simulink model "local_sequencer_harness1"  (R2018b)
settings: Solver=FixedStepDiscrete  StartTime=0  StopTime=8  FixedStep=1  RelTol=1e-3
undefined symbols (not defined in the file or in its folder): eof, sigbuilder_block, sldvsubsys, StateFlowModeType
libraries: sldvlib x21, simulink x6, hdlsllib x4
(part 1 of 2)
settings Model: SldvGeneratedHarnessModel=TestUnitModel=local_sequencer|  Creator=hiterd  LastModifiedBy=gauthamsm
settings DataIOCC: SaveFormat=StructureWithTime
settings OptimizationCC: BlockReduction=off  ConditionallyExecuteInputs=off  DefaultParameterBehavior=Inlined  ExpressionFolding=off
settings DebuggingCC: InheritedTsInSrcMsg=none  LibraryContextMissingDiagnostic=none
settings SFSimCC: SimUseLocalCustomCode=off
settings RTWCC: RTWUseLocalCustomCode=off
settings ConfigComp: DVMode=PropertyProving  DVModelCoverageObjectives=MCDC  DVTestSuiteOptimization=CombinedObjectives (Nonlinear Extended)  DVDetectOutOfBounds=on  DVSaveExpectedOutput=on  DVDisplayReport=off

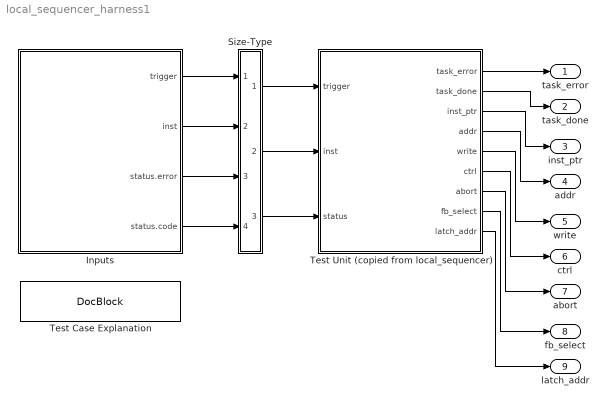
== system local_sequencer_harness1 ==
  Inputs : Subsystem  Tag=STV Subsys  LoadFcn=sigbuilder_block('load',[50 50 520 400 ]);  StartFcn=sigbuilder_block('start');  StopFcn=sigbuilder_block('stop');  ClipboardFcn=sigbuilder_block('clipboard');  mask(Sigbuilder block){tuvar=[0:10]}
      mask init:
      | if ~strcmp(get_param(bdroot(gcb),'SimulationStatus'),'stopped'),tuvar = sigbuilder_block('maskInit'); end
      settings: CopyFcn=sigbuilder_block('copy');  DeleteFcn=sigbuilder_block('delete');  ModelCloseFcn=sigbuilder_block('modelClose');  PreSaveFcn=sigbuilder_block('preSave');  PauseFcn=sigbuilder_block('pause');  ContinueFcn=sigbuilder_block('continue');  NameChangeFcn=sigbuilder_block('namechange');  OpenFcn=sigbuilder_block('open');  CloseFcn=sigbuilder_block('close');
      mask Display: plot(0, 0, 100, 100,[2, 2, 32, 32, 2], [68, 8, 8, 68, 68],[32, 2], [38, 38], [32, 19, 2],[53, 60, 44], [32, 17, 17, 2],[16, 16, 31, 31]);txt = getActiveGroup(gcbh);text(2, 100, txt,'verticalAlignment', 'top');
  Size-Type : Subsystem
  Test Case Explanation : simulink/Model-Wide Utilities/DocBlock  DocumentType=Text
  Test Unit (copied from local_sequencer) : Subsystem
  task_error : Outport  RequirementInfo={'linktype_rmi_slreq' 'local_sequencer_req.slreqx' '20' 'true' 'ERROR (local_sequencer_req#20)' '' ; 'linktype_rmi_slreq' 'local_sequencer_req.slreqx' '29' 'true' 'Error Signal Service Provided (local_sequencer_req#29)' '' } %GIDa_6eef222e_a01c_4fe0_8b87_beeef317aa57  OutDataTypeStr=boolean
  task_done : Outport  RequirementInfo={'linktype_rmi_slreq' 'local_sequencer_req.slreqx' '19' 'true' 'TASK_DONE (local_sequencer_req#19)' '' ; 'linktype_rmi_slreq' 'local_sequencer_req.slreqx' '30' 'true' 'Task Done Service Provided (local_sequencer_req#30)' '' } %GIDa_6d4806b7_f9de_4eac_b969_3ebe75b1e1cf  Port=2  OutDataTypeStr=boolean
  inst_ptr : Outport  RequirementInfo={'linktype_rmi_slreq' 'local_sequencer_req.slreqx' '32' 'true' 'Instruction Pointer Service Provided (local_sequencer_req#32)' '' } %GIDa_7b08b03b_531f_4ab3_8a58_ea9a3981e577  Port=3  OutDataTypeStr=task_inst_ptr_type
  addr : Outport  RequirementInfo={'linktype_rmi_slreq' 'local_sequencer_req.slreqx' '31' 'true' 'Task Memory Control Service Provided (local_sequencer_req#31)' '' } %GIDa_6cc3cc84_3630_4849_818a_038d439d27b6  Port=4  OutMin=[0]  OutDataTypeStr=task_memory_addr_type
  write : Outport  RequirementInfo={'linktype_rmi_slreq' 'local_sequencer_req.slreqx' '17' 'true' 'WRITE (local_sequencer_req#17)' '' ; 'linktype_rmi_slreq' 'local_sequencer_req.slreqx' '31' 'true' 'Task Memory Control Service Provided (local_sequencer_req#31)' '' } %GIDa_5bef7a76_c2bd_49e5_8166_1c241c27171b  Port=5  OutDataTypeStr=boolean
  ctrl : Outport  RequirementInfo={'linktype_rmi_slreq' 'local_sequencer_req.slreqx' '15' 'true' 'FETCH (local_sequencer_req#15)' '' ; 'linktype_rmi_slreq' 'local_sequencer_req.slreqx' '16' 'true' 'FB_EXECUTE (local_sequencer_req#16)' '' ; 'linktype_rmi_slreq' 'local_sequencer_req.slreqx' '17' 'true' 'WRITE (local_sequencer_req#17)' '' ; 'linktype_rmi_slreq' 'local_sequencer_req.slreqx' '18' 'true' 'FB_DONE (local_sequencer_req#18)' '' } %GIDa_e9a2eb4e_1730_43fc_aa4d_0d480ce4c4e5  Port=6  OutDataTypeStr=boolean
  abort : Outport  RequirementInfo={'linktype_rmi_slreq' 'local_sequencer_req.slreqx' '20' 'true' 'ERROR (local_sequencer_req#20)' '' } %GIDa_377a1d8d_f365_49c2_8f09_411d47a425b6  Port=7  OutDataTypeStr=boolean
  fb_select : Outport  RequirementInfo={'linktype_rmi_slreq' 'local_sequencer_req.slreqx' '33' 'true' 'Function Block Selection Service Provided (local_sequencer_req#33)' '' } %GIDa_773eebd4_072a_4a77_a6f5_8af07ffa45d2  Port=8  OutDataTypeStr=fb_select_type
  latch_addr : Outport  RequirementInfo={} %GIDa_0990d834_66a0_4e94_ab9b_9875cb70122a  Port=9  OutMin=[0]  OutDataTypeStr=boolean
  wires:
  Inputs/1(trigger) -> Size-Type/1(In1)
  Size-Type/1(Out1) -> Test Unit (copied from local_sequencer)/1(trigger)
  Inputs/2(inst) -> Size-Type/2(In2)
  Size-Type/2(Out2) -> Test Unit (copied from local_sequencer)/2(inst)
  Inputs/3(status.error) -> Size-Type/3(In5)
  Inputs/4(status.code) -> Size-Type/4(In6)
  Size-Type/3(Out3) -> Test Unit (copied from local_sequencer)/3(status)
  Test Unit (copied from local_sequencer)/1(task_error) -> task_error/1
  Test Unit (copied from local_sequencer)/2(task_done) -> task_done/1
  Test Unit (copied from local_sequencer)/3(inst_ptr) -> inst_ptr/1
  Test Unit (copied from local_sequencer)/4(addr) -> addr/1
  Test Unit (copied from local_sequencer)/5(write) -> write/1
  Test Unit (copied from local_sequencer)/6(ctrl) -> ctrl/1
  Test Unit (copied from local_sequencer)/7(abort) -> abort/1
  Test Unit (copied from local_sequencer)/8(fb_select) -> fb_select/1
  Test Unit (copied from local_sequencer)/9(latch_addr) -> latch_addr/1

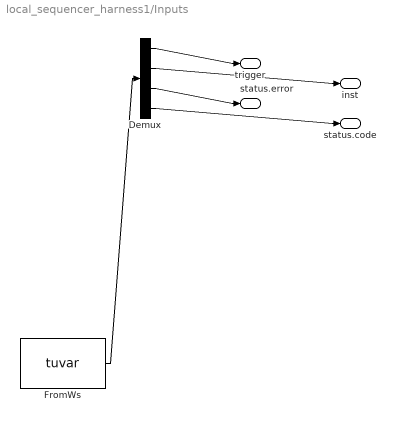
== system local_sequencer_harness1/Inputs ==
  Demux : Demux  Tag=STV Demux
  FromWs : FromWorkspace  Tag=STV FromWs  VariableName=tuvar  SampleTime=0
      SigBuilderData=|
      | dataSet(1).timeRange = [0 7]
      | dataSet(1).name = 'Counterexample 1'
      | dataSet(2).timeRange = [0 8]
      | dataSet(2).name = 'Counterexample 2'
      | sbobj.Name = 'Signal Builder'
      | sbobj.Groups(1).Name = 'Counterexample 1'
      | sbobj.Groups(1).Signals(1).Name = 'trigger'
      | sbobj.Groups(1).Signals(1).XData = [0 1 2 3 4 5 5 6 7]
      | sbobj.Groups(1).Signals(1).YData = [1 1 1 1 1 1 0 0 0]
      | sbobj.Groups(1).Signals(2).Name = 'inst'
      | sbobj.Groups(1).Signals(2).XData = [0 1 2 3 4 5 6 7]
      | sbobj.Groups(1).Signals(2).YData = [2147483646 2147483646 2147483646 2147483646 2147483646 2147483646 2147483646 2147483646]
      | sbobj.Groups(1).Signals(3).Name = 'status.error'
      | sbobj.Groups(1).Signals(3).XData = [0 1 2 3 3 4 5 5 6 7]
      | sbobj.Groups(1).Signals(3).YData = [0 0 0 0 1 1 1 0 0 0]
      | sbobj.Groups(1).Signals(4).Name = 'status.code'
      | sbobj.Groups(1).Signals(4).XData = [0 1 1 2 2 3 3 4 4 5 5 6 6 7]
      | sbobj.Groups(1).Signals(4).YData = [71303169 71303169 8388609 8388609 2227175425 2227175425 2164260864 2164260864 2235564032 2235564032 2239758337 2239758337 96468993 96468993]
      | sbobj.Groups(1).TimeRange = [0 7]
      | sbobj.Groups(2).Name = 'Counterexample 2'
      | sbobj.Groups(2).Signals(1).Name = 'trigger'
      | sbobj.Groups(2).Signals(1).XData = [0 1 2 3 4 5 5 6 7 7 8]
      | sbobj.Groups(2).Signals(1).YData = [1 1 1 1 1 1 0 0 0 1 1]
      | sbobj.Groups(2).Signals(2).Name = 'inst'
      | sbobj.Groups(2).Signals(2).XData = [0 1 2 3 4 5 6 7 8]
      | sbobj.Groups(2).Signals(2).YData = [2147483646 2147483646 2147483646 2147483646 2147483646 2147483646 2147483646 2147483646 2147483646]
      | sbobj.Groups(2).Signals(3).Name = 'status.error'
      | sbobj.Groups(2).Signals(3).XData = [0 1 2 3 3 4 5 5 6 7 8]
      | sbobj.Groups(2).Signals(3).YData = [0 0 0 0 1 1 1 0 0 0 0]
      | sbobj.Groups(2).Signals(4).Name = 'status.code'
      | sbobj.Groups(2).Signals(4).XData = [0 1 1 2 2 3 3 4 4 5 5 6 6 7 7 8]
      | sbobj.Groups(2).Signals(4).YData = [71303169 71303169 8388609 8388609 2227175425 2227175425 2164260865 2164260865 2235564033 2235564033 2239758337 2239758337 2243952640 2243952640 100663297 100663297]
      | sbobj.Groups(2).TimeRange = [0 8]
  trigger : Outport  Tag=STV Outport
  inst : Outport  Tag=STV Outport  Port=2
  status.error : Outport  Tag=STV Outport  Port=3
  status.code : Outport  Tag=STV Outport  Port=4
  wires:
  FromWs/1 -> Demux/1
  Demux/1 -> trigger/1
  Demux/2 -> inst/1
  Demux/3 -> status.error/1
  Demux/4 -> status.code/1

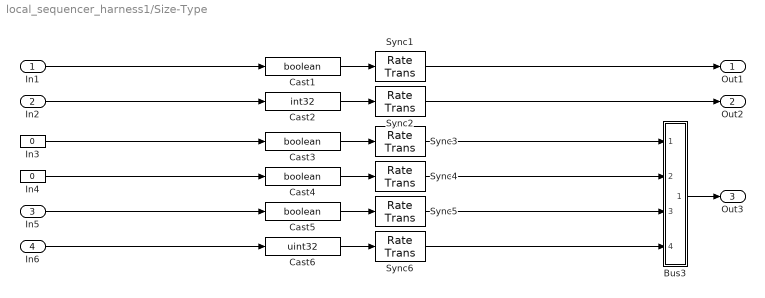
== system local_sequencer_harness1/Size-Type ==
  In1 : Inport
  In2 : Inport  Port=2
  In5 : Inport  Port=3
  In6 : Inport  Port=4
  Bus3 : Subsystem
  Cast{1,3..5} (4 alike) : DataTypeConversion  OutDataTypeStr=boolean  RndMeth=Nearest  SaturateOnIntegerOverflow=on
  Cast2 : DataTypeConversion  OutDataTypeStr=int32  RndMeth=Nearest  SaturateOnIntegerOverflow=on
  Cast6 : DataTypeConversion  OutDataTypeStr=uint32  RndMeth=Nearest  SaturateOnIntegerOverflow=on
  In3 : Constant  Value=0  OutDataTypeStr=double
  In4 : Constant  Value=0  OutDataTypeStr=double
  Sync{1..6} (6 alike) : RateTransition  OutPortSampleTime=[1,0]
  Out1 : Outport
  Out2 : Outport  Port=2
  Out3 : Outport  Port=3
  wires:
  In1/1 -> Cast1/1
  Cast1/1 -> Sync1/1
  Sync1/1 -> Out1/1
  In2/1 -> Cast2/1
  Cast2/1 -> Sync2/1
  Sync2/1 -> Out2/1
  In3/1 -> Cast3/1
  Cast3/1 -> Sync3/1
  In4/1 -> Cast4/1
  Cast4/1 -> Sync4/1
  In5/1 -> Cast5/1
  Cast5/1 -> Sync5/1
  In6/1 -> Cast6/1
  Cast6/1 -> Sync6/1
  Sync3/1 -> Bus3/1(status(1).done)
  Sync4/1 -> Bus3/2(status(1).busy)
  Sync5/1 -> Bus3/3(status(1).error)
  Sync6/1 -> Bus3/4(status(1).code)
  Bus3/1(Out) -> Out3/1

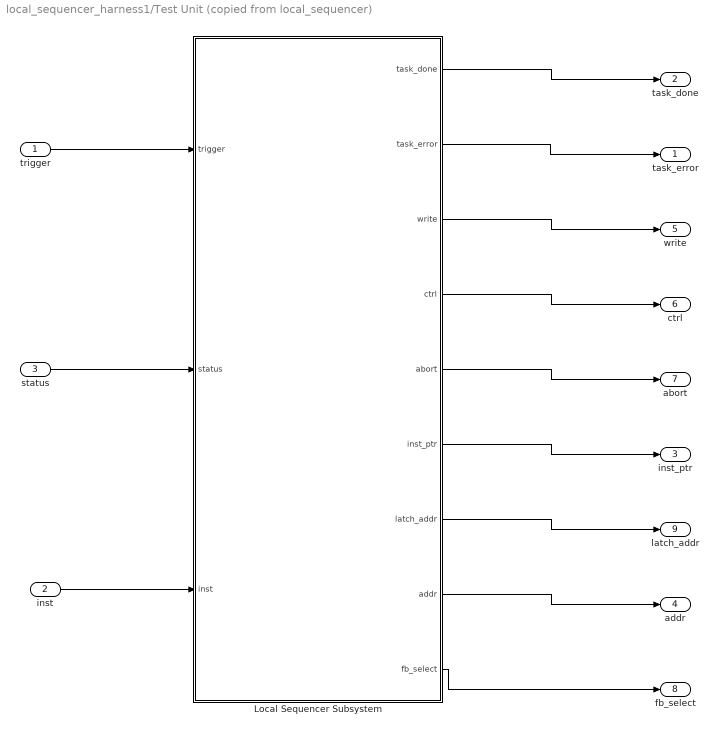
== system local_sequencer_harness1/Test Unit (copied from local_sequencer) ==
  trigger : Inport  RequirementInfo={'linktype_rmi_slreq' 'local_sequencer_req.slreqx' '1' 'true' 'Trigger Service Received (local_sequencer_req#1)' '' } %GIDa_ee1d0688_7702_4e59_8607_409a267b03c8  OutDataTypeStr=boolean  SampleTime=1
  inst : Inport  RequirementInfo={'linktype_rmi_slreq' 'local_sequencer_req.slreqx' '2' 'true' 'Instruction Service Received (local_sequencer_req#2)' '' } %GIDa_47f0b591_29ce_4c3a_8458_22a20f7cfe60  Port=2  OutDataTypeStr=task_inst_data_type  SampleTime=1
  status : Inport  RequirementInfo={'linktype_rmi_slreq' 'local_sequencer_req.slreqx' '3' 'true' 'Function Block Status Service Received (local_sequencer_req#3)' '' } %GIDa_5f43f148_b0c6_4574_8c0e_1a7e8a450581  Port=3  OutDataTypeStr=Bus: fb_status  SampleTime=1
  Local Sequencer Subsystem : Subsystem  RequirementInfo={} %GIDa_1bf9c4de_d1bc_41bc_89dd_bd5a58f40b8b
  task_error : Outport  RequirementInfo={'linktype_rmi_slreq' 'local_sequencer_req.slreqx' '20' 'true' 'ERROR (local_sequencer_req#20)' '' ; 'linktype_rmi_slreq' 'local_sequencer_req.slreqx' '29' 'true' 'Error Signal Service Provided (local_sequencer_req#29)' '' } %GIDa_20f58596_03f6_49ea_9ef8_6cf8984f0cae  OutDataTypeStr=boolean
  task_done : Outport  RequirementInfo={'linktype_rmi_slreq' 'local_sequencer_req.slreqx' '19' 'true' 'TASK_DONE (local_sequencer_req#19)' '' ; 'linktype_rmi_slreq' 'local_sequencer_req.slreqx' '30' 'true' 'Task Done Service Provided (local_sequencer_req#30)' '' } %GIDa_bf8ce283_f71f_479c_b035_26f3616a3704  Port=2  OutDataTypeStr=boolean
  inst_ptr : Outport  RequirementInfo={'linktype_rmi_slreq' 'local_sequencer_req.slreqx' '32' 'true' 'Instruction Pointer Service Provided (local_sequencer_req#32)' '' } %GIDa_0f6bf1a4_d050_45ca_8bf8_3a42e5078f97  Port=3  OutDataTypeStr=task_inst_ptr_type
  addr : Outport  RequirementInfo={'linktype_rmi_slreq' 'local_sequencer_req.slreqx' '31' 'true' 'Task Memory Control Service Provided (local_sequencer_req#31)' '' } %GIDa_98fe4c2c_df0f_4e0e_8fd6_d95b2a2e6c87  Port=4  OutMin=[0]  OutDataTypeStr=task_memory_addr_type
  write : Outport  RequirementInfo={'linktype_rmi_slreq' 'local_sequencer_req.slreqx' '17' 'true' 'WRITE (local_sequencer_req#17)' '' ; 'linktype_rmi_slreq' 'local_sequencer_req.slreqx' '31' 'true' 'Task Memory Control Service Provided (local_sequencer_req#31)' '' } %GIDa_17540029_023b_4499_94ff_6577575a4c02  Port=5  OutDataTypeStr=boolean
  ctrl : Outport  RequirementInfo={'linktype_rmi_slreq' 'local_sequencer_req.slreqx' '15' 'true' 'FETCH (local_sequencer_req#15)' '' ; 'linktype_rmi_slreq' 'local_sequencer_req.slreqx' '16' 'true' 'FB_EXECUTE (local_sequencer_req#16)' '' ; 'linktype_rmi_slreq' 'local_sequencer_req.slreqx' '17' 'true' 'WRITE (local_sequencer_req#17)' '' ; 'linktype_rmi_slreq' 'local_sequencer_req.slreqx' '18' 'true' 'FB_DONE (local_sequencer_req#18)' '' } %GIDa_b953f4cf_75e3_49f5_957d_136b7d9f114f  Port=6  OutDataTypeStr=boolean
  abort : Outport  RequirementInfo={'linktype_rmi_slreq' 'local_sequencer_req.slreqx' '20' 'true' 'ERROR (local_sequencer_req#20)' '' } %GIDa_64b414b4_42fd_4a02_80e3_9b85f133adaf  Port=7  OutDataTypeStr=boolean
  fb_select : Outport  RequirementInfo={'linktype_rmi_slreq' 'local_sequencer_req.slreqx' '33' 'true' 'Function Block Selection Service Provided (local_sequencer_req#33)' '' } %GIDa_ebf60c88_1429_4d3a_8715_399b1e400c0c  Port=8  OutDataTypeStr=fb_select_type
  latch_addr : Outport  RequirementInfo={} %GIDa_5b9c4f65_97de_40d7_b2b2_078d0fae9703  Port=9  OutMin=[0]  OutDataTypeStr=boolean
  wires:
  trigger/1 -> Local Sequencer Subsystem/1(trigger)
  status/1 -> Local Sequencer Subsystem/2(status)
  inst/1 -> Local Sequencer Subsystem/3(inst)
  Local Sequencer Subsystem/1(task_done) -> task_done/1
  Local Sequencer Subsystem/2(task_error) -> task_error/1
  Local Sequencer Subsystem/3(write) -> write/1
  Local Sequencer Subsystem/4(ctrl) -> ctrl/1
  Local Sequencer Subsystem/5(abort) -> abort/1
  Local Sequencer Subsystem/6(inst_ptr) -> inst_ptr/1
  Local Sequencer Subsystem/7(latch_addr) -> latch_addr/1
  Local Sequencer Subsystem/8(addr) -> addr/1
  Local Sequencer Subsystem/9(fb_select) -> fb_select/1

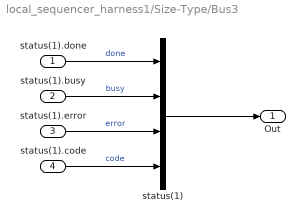
== system local_sequencer_harness1/Size-Type/Bus3 ==
  status(1).done : Inport
  status(1).busy : Inport  Port=2
  status(1).error : Inport  Port=3
  status(1).code : Inport  Port=4
  status(1) : BusCreator  Inputs=4  OutDataTypeStr=Bus: fb_status
  Out : Outport
  wires:
  status(1).done/1 -> status(1)/1  "done"
  status(1).busy/1 -> status(1)/2  "busy"
  status(1).error/1 -> status(1)/3  "error"
  status(1).code/1 -> status(1)/4  "code"
  status(1)/1 -> Out/1

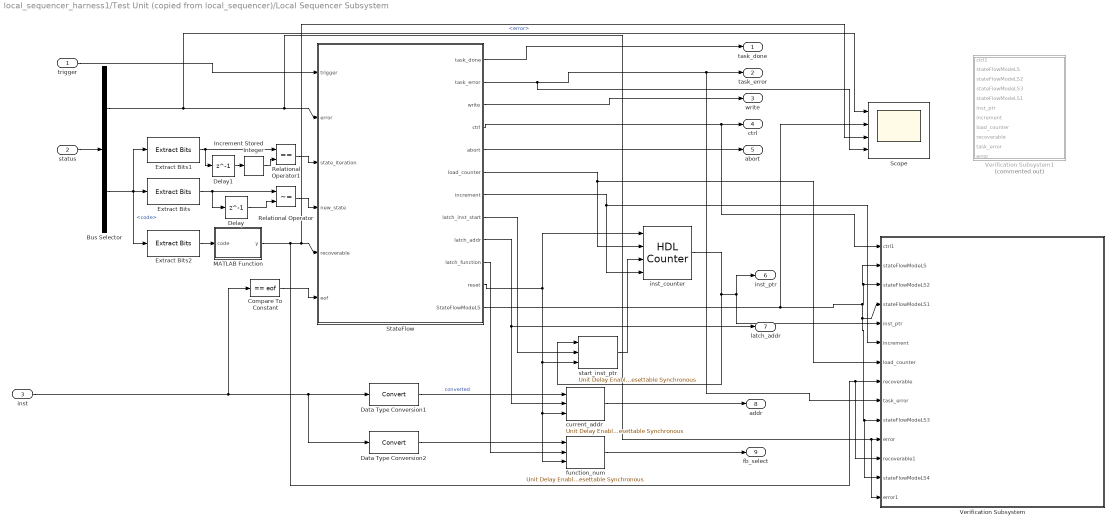
== system local_sequencer_harness1/Test Unit (copied from local_sequencer)/Local Sequencer Subsystem ==
  trigger : Inport  RequirementInfo={} %GIDa_667813c0_2ce9_40e6_9192_d23a19fa8e60
  status : Inport  RequirementInfo={} %GIDa_9f922e78_e05f_4ac9_a2b3_e973c3d7ad29  Port=2
  inst : Inport  RequirementInfo={} %GIDa_4c36c994_e89b_42c1_b8ba_4a193efc4b8e  Port=3
  Bus Selector : BusSelector  RequirementInfo={} %GIDa_79b6253a_0006_455f_9c58_eb6258196a1d  OutputSignals=error,code
  Compare To Constant : simulink/Logic and Bit Operations/Compare To Constant  RequirementInfo={'linktype_rmi_slreq' 'local_sequencer_req.slreqx' '7' 'true' 'End of File Determination (local_sequencer_req#7)' '' } %GIDa_d4bef37c_6deb_46bc_b5d5_b2c59b772020  relop===  const=eof  OutDataTypeStr=boolean
  Data Type Conversion1 : DataTypeConversion  RequirementInfo={'linktype_rmi_slreq' 'local_sequencer_req.slreqx' '34' 'true' 'Conversion of Data Input (local_sequencer_req#34)' '' } %GIDa_3a8a9ada_8e73_438c_a14d_fd8a1bd1786e
  Data Type Conversion2 : DataTypeConversion  RequirementInfo={'linktype_rmi_slreq' 'local_sequencer_req.slreqx' '34' 'true' 'Conversion of Data Input (local_sequencer_req#34)' '' } %GIDa_a57cdd45_237b_4637_96ce_ae33a3fb69d7
  Delay : Delay  RequirementInfo={'linktype_rmi_slreq' 'local_sequencer_req.slreqx' '5' 'true' 'Super State Change Detection (local_sequencer_req#5)' '' } %GIDa_45c36634_f8e4_4883_a8b8_e675ae30925e  DelayLength=1
  Delay1 : Delay  RequirementInfo={'linktype_rmi_slreq' 'local_sequencer_req.slreqx' '4' 'true' 'Super State Iteration Detection (local_sequencer_req#4)' '' } %GIDa_6506c89b_1702_47b1_a15e_211730d3d040  DelayLength=1
  Extract Bits : simulink/Logic and Bit Operations/Extract Bits  RequirementInfo={'linktype_rmi_slreq' 'local_sequencer_req.slreqx' '5' 'true' 'Super State Change Detection (local_sequencer_req#5)' '' } %GIDa_a09b6f6c_4604_4977_b275_4d844021750a  bitsToExtract=Range starting with most significant bit  numBits=4  bitIdxRange=[0 7]  outScalingMode=Treat bit field as an integer
      settings: SourceProductName=Simulink
  Extract Bits1 : simulink/Logic and Bit Operations/Extract Bits  RequirementInfo={'linktype_rmi_slreq' 'local_sequencer_req.slreqx' '4' 'true' 'Super State Iteration Detection (local_sequencer_req#4)' '' } %GIDa_e2105eee_930a_4cdf_b252_ae460803f0fd  bitsToExtract=Range of bits  numBits=4  bitIdxRange=[22 27]  outScalingMode=Treat bit field as an integer
      settings: SourceProductName=Simulink
  Extract Bits2 : simulink/Logic and Bit Operations/Extract Bits  RequirementInfo={'linktype_rmi_slreq' 'local_sequencer_req.slreqx' '6' 'true' 'Error Recovery Determination (local_sequencer_req#6)' '' } %GIDa_b560e2a3_a7f1_476c_8b2a_ffbd10a00e53  bitsToExtract=Range ending with least significant bit  numBits=22  bitIdxRange=[22 27]  outScalingMode=Treat bit field as an integer
      settings: SourceProductName=Simulink
  Increment Stored Integer : simulink/Additional Math & Discrete/Additional Math: Increment - Decrement/Increment Stored Integer  RequirementInfo={'linktype_rmi_slreq' 'local_sequencer_req.slreqx' '4' 'true' 'Super State Iteration Detection (local_sequencer_req#4)' '' } %GIDa_7ee8b49c_7e9e_43d6_94a5_684ad1a7ac3c
      settings: SourceProductName=Simulink
  MATLAB Function : MATLAB Function  RequirementInfo={'linktype_rmi_slreq' 'local_sequencer_req.slreqx' '6' 'true' 'Error Recovery Determination (local_sequencer_req#6)' '' } %GIDa_66948775_d3bd_4a51_9bc7_416a7d662e0f  TreatAsAtomicUnit=on
  Relational Operator : RelationalOperator  RequirementInfo={'linktype_rmi_slreq' 'local_sequencer_req.slreqx' '5' 'true' 'Super State Change Detection (local_sequencer_req#5)' '' } %GIDa_e58a5a39_9204_403d_bf5d_efec21faad89  Operator=~=  OutDataTypeStr=boolean  RndMeth=Nearest
  Relational Operator1 : RelationalOperator  RequirementInfo={'linktype_rmi_slreq' 'local_sequencer_req.slreqx' '4' 'true' 'Super State Iteration Detection (local_sequencer_req#4)' '' } %GIDa_773bf6c2_074e_418a_ba1a_320df8c963b4  Operator===  OutDataTypeStr=boolean  RndMeth=Nearest
  Scope : Scope  NumInputPorts=4
      settings: RequirementInfo={} %GIDa_a31c3830_a24c_4eea_be79_7702308a54d4
  StateFlow : Stateflow chart  RequirementInfo={'linktype_rmi_slreq' 'local_sequencer_req.slreqx' '12' 'true' 'Controller Super States (local_sequencer_req#12)' '' } %GIDa_024dda5f_4f1f_4977_87f0_8beb7680ab0a  TreatAsAtomicUnit=on
  Verification Subsystem : Subsystem  Tag=VerificationSubsystem  RequirementInfo={} %GIDa_838dcf04_7b59_4d43_9019_59a44524fb9a  DisableCoverage=on  LoadFcn=sldvsubsys('check')  TreatAsAtomicUnit=on  SimViewingDevice=on  mask(VerificationSubsystem){}
      mask init:
      | sldvsubsys('maskInit');
      settings: CopyFcn=sldvsubsys('copy');  OpenFcn=open_system(gcb,'force');
      settings: PreSaveFcn=|
      | set_param(gcb,'SimViewingDevice','on');
      | sldvsubsys('check');
      mask Help: helpview(fullfile(docroot,'toolbox','sldv','sldv.map'),'verificationsubsystem')
      mask Display: image(imread('sldvicon_versubsys.png','BackGroundColor',[1 1 1]),'center');
  Verification Subsystem1 : Subsystem  Tag=VerificationSubsystem  RequirementInfo={} %GIDa_73cb3161_c03e_414d_bb3b_35ff3da55f89  Commented=on  DisableCoverage=on  LoadFcn=sldvsubsys('check')  TreatAsAtomicUnit=on  SimViewingDevice=on  mask(VerificationSubsystem){}
      mask init:
      | sldvsubsys('maskInit');
      settings: CopyFcn=sldvsubsys('copy');  OpenFcn=open_system(gcb,'force');
      settings: PreSaveFcn=|
      | set_param(gcb,'SimViewingDevice','on');
      | sldvsubsys('check');
      mask Help: helpview(fullfile(docroot,'toolbox','sldv','sldv.map'),'verificationsubsystem')
      mask Display: image(imread('sldvicon_versubsys.png','BackGroundColor',[1 1 1]),'center');
  current_addr : hdlsllib/Discrete/Unit Delay Enabled Resettable Synchronous  RequirementInfo={'linktype_rmi_slreq' 'local_sequencer_req.slreqx' '11' 'true' 'Current Address Register (local_sequencer_req#11)' '' } %GIDa_563c094f_6702_4153_896a_e0e79255b215  InitialCondition=0  SampleTime=-1
      settings: SourceProductName=HDL Coder  SourceProductBaseCode=HD
  function_num : hdlsllib/Discrete/Unit Delay Enabled Resettable Synchronous  RequirementInfo={'linktype_rmi_slreq' 'local_sequencer_req.slreqx' '8' 'true' 'Function Number Register (local_sequencer_req#8)' '' } %GIDa_966114bc_cb8e_417e_b29d_e0445db8d5d9  InitialCondition=0  SampleTime=-1
      settings: SourceProductName=HDL Coder  SourceProductBaseCode=HD
  inst_counter : hdlsllib/Sources/HDL Counter  RequirementInfo={'linktype_rmi_slreq' 'local_sequencer_req.slreqx' '10' 'true' 'Instruction Counter (local_sequencer_req#10)' '' } %GIDa_defabc86_250d_4a18_b0b1_c3bf708ae8ef  CountType=Free running  CountInit=0  CountStep=1  CountMax=25  CountFromType=Initial value  CountFrom=0  CountResetPort=on  CountLoadPort=on  CountEnbPort=on  CountDirPort=off  CountDataType=Unsigned  CountWordLen=32  CountFracLen=0  CountSampTime=1
      settings: SourceProductBaseCode=HD
  start_inst_ptr : hdlsllib/Discrete/Unit Delay Enabled Resettable Synchronous  RequirementInfo={'linktype_rmi_slreq' 'local_sequencer_req.slreqx' '9' 'true' 'Start Instruction Pointer Register (local_sequencer_req#9)' '' } %GIDa_aaa9132d_cf81_4cca_ae88_9fa712b7ddec  InitialCondition=0  SampleTime=-1
      settings: SourceProductName=HDL Coder  SourceProductBaseCode=HD
  task_done : Outport  RequirementInfo={} %GIDa_60169851_d1f8_4054_83f8_3a56cf840165
  task_error : Outport  RequirementInfo={} %GIDa_5efbc127_0fad_4743_88d8_48387155e0aa  Port=2
  write : Outport  RequirementInfo={} %GIDa_a41ba5f4_8ba0_4949_8978_bbcfcaae8be3  Port=3
  ctrl : Outport  RequirementInfo={} %GIDa_2ac6603d_f9d3_4fa3_8391_63091cb403f2  Port=4
  abort : Outport  RequirementInfo={} %GIDa_76ad2b85_6a3f_4b60_a575_66190255e4d6  Port=5
  inst_ptr : Outport  RequirementInfo={} %GIDa_93e88be8_92b1_4795_b847_f82d81a6b850  Port=6
  latch_addr : Outport  RequirementInfo={} %GIDa_7a272877_8229_44a5_bbef_389013ad2e48  Port=7
  addr : Outport  RequirementInfo={} %GIDa_458cb3b4_2944_4610_af65_cc656e5cadff  Port=8
  fb_select : Outport  RequirementInfo={} %GIDa_946b26ee_232b_42dd_b12d_200ca52a7a09  Port=9
  wires:
  StateFlow/12(StateFlowModeLS) -> Verification Subsystem/2(stateFlowModeLS), Verification Subsystem/3(stateFlowModeLS2), Verification Subsystem/4(stateFlowModeLS1), Verification Subsystem/10(stateFlowModeLS3), Verification Subsystem/13(stateFlowModeLS4), Scope/2
  StateFlow/3(write) -> write/1
  current_addr/1 -> addr/1
  StateFlow/4(ctrl) -> ctrl/1, Verification Subsystem/1(ctrl1)
  StateFlow/1(task_done) -> task_done/1
  trigger/1 -> StateFlow/1(trigger)
  Extract Bits/1 -> Delay/1, Relational Operator/1
  MATLAB Function/1(y) -> StateFlow/5(recoverable), Scope/3, Verification Subsystem/8(recoverable), Verification Subsystem/12(recoverable1)
  StateFlow/10(latch_function) -> function_num/2
  Data Type Conversion2/1 -> function_num/1
  Relational Operator1/1 -> StateFlow/3(state_iteration)
  Delay/1 -> Relational Operator/2
  StateFlow/2(task_error) -> task_error/1, Verification Subsystem/9(task_error), Scope/4
  function_num/1 -> fb_select/1
  inst/1 -> Compare To Constant/1, Data Type Conversion2/1, Data Type Conversion1/1
  Compare To Constant/1 -> StateFlow/6(eof)
  Relational Operator/1 -> StateFlow/4(new_state)
  Bus Selector/1 -> StateFlow/2(error), Verification Subsystem/11(error), Verification Subsystem/14(error1), Scope/1  "<error>"
  inst_counter/1 -> start_inst_ptr/1, inst_ptr/1, Verification Subsystem/5(inst_ptr)
  Increment Stored Integer/1 -> Relational Operator1/2
  Delay1/1 -> Increment Stored Integer/1
  StateFlow/5(abort) -> abort/1
  Extract Bits1/1 -> Relational Operator1/1, Delay1/1
  Extract Bits2/1 -> MATLAB Function/1(code)
  Bus Selector/2 -> Extract Bits/1, Extract Bits1/1, Extract Bits2/1  "<code>"
  StateFlow/6(load_counter) -> inst_counter/2, Verification Subsystem/7(load_counter)
  StateFlow/11(reset) -> inst_counter/1, start_inst_ptr/3, current_addr/3, function_num/3
  start_inst_ptr/1 -> inst_counter/3
  Data Type Conversion1/1 -> current_addr/1  "converted"
  status/1 -> Bus Selector/1
  StateFlow/7(increment) -> inst_counter/4, Verification Subsystem/6(increment)
  StateFlow/8(latch_inst_start) -> start_inst_ptr/2
  StateFlow/9(latch_addr) -> current_addr/2, latch_addr/1

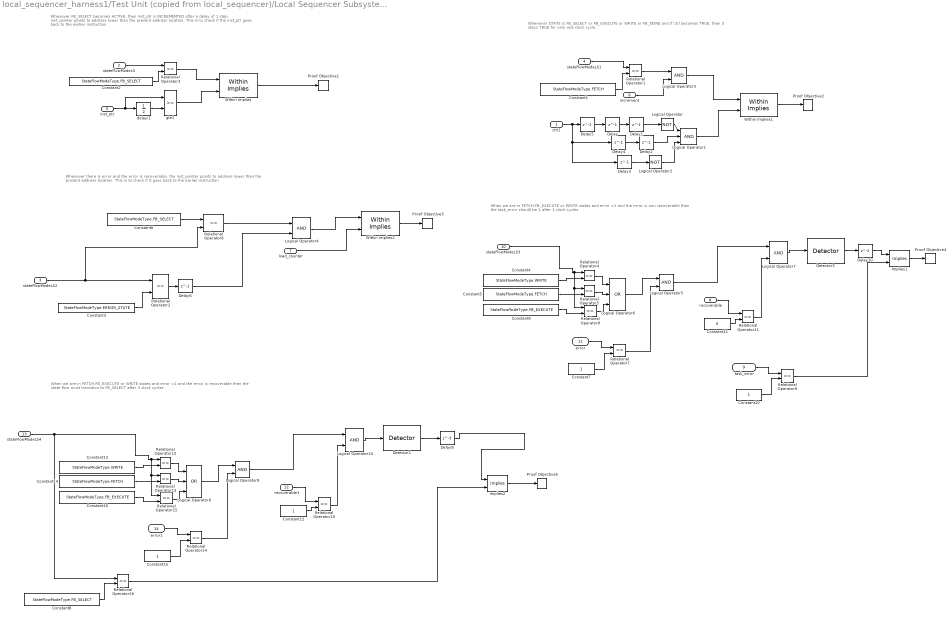
== system local_sequencer_harness1/Test Unit (copied from local_sequencer)/Local Sequencer Subsystem/Verification Subsystem ==
  note: When we are in FETCH,FB_EXECUTE or WRITE states and error =1 and the error is
      | recoverable then the state flow must transition to FB_SELECT after 3 clock cycles
  note: When we are in FETCH,FB_EXECUTE or WRITE states and error =1 and the error is non
      | recoverable then the task_error should be 1 after 2 clock cycles
  note: Whenever there is error and the error is recoverable, the inst_pointer points to address lower than the present address location. This is to check if it goes back to the earlier instruction
  note: Whenever STATE is FB_SELECT or FB_EXECUTE or WRITE or FB_DONE and if ctrl becomes TRUE, then it stays TRUE for only one clock cycle.
  note: Whenever FB_SELECT becomes ACTIVE, then inst_ptr is INCREMENTED after a delay of 1 step. inst_pointer points to address lower than the present address location. This is to check if the inst_ptr goes back to the earlier instruction
  ctrl1 : Inport  RequirementInfo={} %GIDa_2aa84e78_773c_4371_ae03_7363d7f38b64
  stateFlowModeLS : Inport  RequirementInfo={} %GIDa_cd1fa512_6795_43c1_a135_e70df5671345  Port=2  OutDataTypeStr=Enum: StateFlowModeType
  stateFlowModeLS2 : Inport  RequirementInfo={} %GIDa_3976201f_7908_44e8_8b3d_db7ce0af8161  Port=3  OutDataTypeStr=Enum: StateFlowModeType
  stateFlowModeLS1 : Inport  RequirementInfo={} %GIDa_58db11b1_1192_4008_8626_1d311f41fd79  Port=4  OutDataTypeStr=Enum: StateFlowModeType
  inst_ptr : Inport  RequirementInfo={} %GIDa_2b709768_3968_4a77_850c_0663ae289538  Port=5
  increment : Inport  RequirementInfo={} %GIDa_12b0bac8_6436_470f_99c5_ea1d75505bb8  Port=6
  load_counter : Inport  RequirementInfo={} %GIDa_d9eb1b57_669b_4c68_bafa_0f99cb4b8103  Port=7
  recoverable : Inport  RequirementInfo={} %GIDa_e4625633_5461_41a2_94bc_72442730136b  Port=8
  task_error : Inport  RequirementInfo={} %GIDa_cec4d3ba_40cf_4886_86fe_07ac90cae5b8  Port=9
  stateFlowModeLS3 : Inport  RequirementInfo={} %GIDa_c7061a7e_edfd_4dbe_80c8_d50c8470702e  Port=10  OutDataTypeStr=Enum: StateFlowModeType
  error : Inport  RequirementInfo={} %GIDa_b8bf48eb_8eb6_416e_ac24_17b4a0747917  Port=11
  recoverable1 : Inport  RequirementInfo={} %GIDa_6e7cca76_8046_47a7_bf72_a71fcb7542f0  Port=12
  stateFlowModeLS4 : Inport  RequirementInfo={} %GIDa_78b59d9b_505a_48a0_9be0_3dce6eb33108  Port=13  OutDataTypeStr=Enum: StateFlowModeType
  error1 : Inport  RequirementInfo={} %GIDa_60759bef_da0f_4b65_ab82_243b85aad350  Port=14
  Constant1 : Constant  RequirementInfo={} %GIDa_2f9b468e_86d5_4e67_b9d8_8570e8207cb9  Value=StateFlowModeType.FETCH
  Constant10 : Constant  RequirementInfo={} %GIDa_67375268_cc36_4cef_9a35_4af1b0917351
  Constant11 : Constant  RequirementInfo={} %GIDa_d249d429_5dab_46a5_ae30_b70515e1066b  Value=0
  Constant12 : Constant  RequirementInfo={} %GIDa_5e4e935c_c05b_470f_a371_33978611d8fb
  Constant13 : Constant  RequirementInfo={} %GIDa_253d0253_5ab4_4aa5_8c7d_2511dde3576a  Value=StateFlowModeType.WRITE
  Constant14 : Constant  RequirementInfo={} %GIDa_27c3072a_ad64_4193_8e57_068ee4e66af4  Value=StateFlowModeType.FETCH
  Constant15 : Constant  RequirementInfo={} %GIDa_3e0e1f5f_6b74_4bf1_a744_9088ebb3dfc4
  Constant16 : Constant  RequirementInfo={} %GIDa_fa8efd79_c799_4a6f_bdb6_1ef59b41cd93  Value=StateFlowModeType.FB_EXECUTE
  Constant2 : Constant  RequirementInfo={} %GIDa_5cb0de8b_a4d2_44b1_bb00_25cedf8883be  Value=StateFlowModeType.FB_SELECT
  Constant3 : Constant  RequirementInfo={} %GIDa_4c250295_da12_4c27_8ee3_9a2df8860d79  Value=StateFlowModeType.ERROR_STATE
  Constant4 : Constant  RequirementInfo={} %GIDa_2a0a2a41_61dc_4491_be58_822443834d8e  Value=StateFlowModeType.WRITE
  Constant5 : Constant  RequirementInfo={} %GIDa_362bda9a_a883_4331_93da_040566b8034c  Value=StateFlowModeType.FETCH
  Constant6 : Constant  RequirementInfo={} %GIDa_80f926aa_74f9_438f_a7de_40768c0b7c3b  Value=StateFlowModeType.FB_SELECT
  Constant7 : Constant  RequirementInfo={} %GIDa_bc8b03f5_f384_4a51_be3b_76328105cdb5
  Constant8 : Constant  RequirementInfo={} %GIDa_9b5bf724_cca9_4760_8981_bb49b685bd29  Value=StateFlowModeType.FB_SELECT
  Constant9 : Constant  RequirementInfo={} %GIDa_6af35a12_229c_4180_8d91_2e416acf6d9d  Value=StateFlowModeType.FB_EXECUTE
  Delay : Delay  RequirementInfo={} %GIDa_ce1a188c_ad47_4410_aca7_c02cd954dce1  DelayLength=1  InitialCondition=0
  Delay1 : Delay  RequirementInfo={} %GIDa_1362c001_f3eb_4d49_bb9c_0e94ad972754  DelayLength=1  InitialCondition=0
  Delay10 : Delay  RequirementInfo={} %GIDa_f01116f0_a0ee_44c9_b379_c02e42b855df  InitialCondition=0
  Delay2 : Delay  RequirementInfo={} %GIDa_1d4055f3_627a_43d5_8e73_8811762443c8  DelayLength=1  InitialCondition=0
  Delay3 : Delay  RequirementInfo={} %GIDa_ff1dd165_ed2d_4858_8b39_a6cd76526871  DelayLength=1  InitialCondition=0
  Delay4 : Delay  RequirementInfo={} %GIDa_c44a1d18_3025_443b_b4c5_471a8ae38f90  DelayLength=1  InitialCondition=0
  Delay5 : Delay  RequirementInfo={} %GIDa_9d77ba82_1771_4fe8_9992_2c0506f2e4b3  DelayLength=1  InitialCondition=0
  Delay6 : Delay  RequirementInfo={} %GIDa_71ec1c03_be14_4fbb_8dbf_80ce0c9cafb7  DelayLength=1  InitialCondition=0
  Delay8 : Delay  RequirementInfo={} %GIDa_c14d562a_418c_4025_9036_cae0ced13188  DelayLength=3  InitialCondition=0
  Detector1 : sldvlib/Temporal Operators/Detector  RequirementInfo={} %GIDa_8af342df_2d87_4d05_b53f_57649a8bece8  reset=off  typ=Synchronized  in_hold=1  delay=0  out_hold=5
      settings: SourceProductName=Simulink Design Verifier  SourceProductBaseCode=DV
  Detector3 : sldvlib/Temporal Operators/Detector  RequirementInfo={} %GIDa_24b06946_3181_402f_85ff_b2b774b0b6eb  reset=off  typ=Synchronized  in_hold=1  delay=0  out_hold=5
      settings: SourceProductName=Simulink Design Verifier  SourceProductBaseCode=DV
  Implies1 : sldvlib/Verification Utilities/Implies  RequirementInfo={} %GIDa_1c89ca27_fa5c_41ad_b908_4e82d2b3e8af
      settings: SourceProductName=Simulink Design Verifier  SourceProductBaseCode=DV
  Implies2 : sldvlib/Verification Utilities/Implies  RequirementInfo={} %GIDa_cbb2abe0_215a_4d24_ad95_12f29e4fb3c4
      settings: SourceProductName=Simulink Design Verifier  SourceProductBaseCode=DV
  Logical Operator : Logic  RequirementInfo={} %GIDa_61ff7ee5_b755_4f1a_91d7_94c52c251ca9  Operator=NOT  AllPortsSameDT=off  OutDataTypeStr=boolean
  Logical Operator1 : Logic  RequirementInfo={} %GIDa_3846ab15_8dd9_4095_b066_9fbc2776fd2e  Inputs=3  AllPortsSameDT=off  OutDataTypeStr=boolean
  Logical Operator10 : Logic  RequirementInfo={} %GIDa_b068508d_63f7_4024_a118_473cbfd4dbe4  AllPortsSameDT=off  OutDataTypeStr=boolean
  Logical Operator2 : Logic  RequirementInfo={} %GIDa_dc10462a_cf28_4017_82d4_4c6ffab9c4b8  Operator=NOT  AllPortsSameDT=off  OutDataTypeStr=boolean
  Logical Operator3 : Logic  RequirementInfo={} %GIDa_80b61834_e5e1_4893_b336_050aa4a3ce76  AllPortsSameDT=off  OutDataTypeStr=boolean
  Logical Operator4 : Logic  RequirementInfo={} %GIDa_3e32758b_ac4a_4dd0_b065_fe585041840a  AllPortsSameDT=off  OutDataTypeStr=boolean
  Logical Operator5 : Logic  RequirementInfo={} %GIDa_682725ea_3691_4e10_bf23_17cc8cf0e81c  AllPortsSameDT=off  OutDataTypeStr=boolean
  Logical Operator6 : Logic  RequirementInfo={} %GIDa_1a223ff8_058f_4edb_b86b_84cde330ac7a  Operator=OR  Inputs=3  AllPortsSameDT=off  OutDataTypeStr=boolean
  Logical Operator7 : Logic  RequirementInfo={} %GIDa_75707b2c_6c6f_4edb_b2e7_a30f65390c2f  AllPortsSameDT=off  OutDataTypeStr=boolean
  Logical Operator8 : Logic  RequirementInfo={} %GIDa_911bdfc3_0d8b_45dd_88b7_061381ed9f8d  AllPortsSameDT=off  OutDataTypeStr=boolean
  Logical Operator9 : Logic  RequirementInfo={} %GIDa_70ebfe4b_f92b_47a5_8eb3_0e675cff94de  Operator=OR  Inputs=3  AllPortsSameDT=off  OutDataTypeStr=boolean
  Proof Objective1 : sldvlib/Objectives and Constraints/Proof Objective  RequirementInfo={} %GIDa_7112df57_b338_4d19_9635_c3797f705c7b  enabled=on  customAVTBlockType=Proof Objective  intervals=true  dispValues=on  outEnabled=off  enableStopSim=off
      settings: AttributesFormatString=%<intervals>  SourceProductName=Simulink Design Verifier  SourceProductBaseCode=DV
  Proof Objective2 : sldvlib/Objectives and Constraints/Proof Objective  RequirementInfo={} %GIDa_4dbc438c_3680_4936_b3eb_536ccf53019f  enabled=on  customAVTBlockType=Proof Objective  intervals=true  dispValues=on  outEnabled=off  enableStopSim=off
      settings: AttributesFormatString=%<intervals>  SourceProductName=Simulink Design Verifier  SourceProductBaseCode=DV
  Proof Objective3 : sldvlib/Objectives and Constraints/Proof Objective  RequirementInfo={} %GIDa_0aa2b519_c2b4_452d_a934_518c9f2c2a78  enabled=on  customAVTBlockType=Proof Objective  intervals=true  dispValues=on  outEnabled=off  enableStopSim=off
      settings: AttributesFormatString=%<intervals>  SourceProductName=Simulink Design Verifier  SourceProductBaseCode=DV
  Proof Objective4 : sldvlib/Objectives and Constraints/Proof Objective  RequirementInfo={} %GIDa_251bef15_81a8_4130_b8c1_53605189bafa  enabled=on  customAVTBlockType=Proof Objective  intervals=true  dispValues=on  outEnabled=off  enableStopSim=off
      settings: AttributesFormatString=%<intervals>  SourceProductName=Simulink Design Verifier  SourceProductBaseCode=DV
  Proof Objective5 : sldvlib/Objectives and Constraints/Proof Objective  RequirementInfo={} %GIDa_55075087_b162_4d88_844f_d5bd540903c3  enabled=on  customAVTBlockType=Proof Objective  intervals=true  dispValues=on  outEnabled=off  enableStopSim=off
      settings: AttributesFormatString=%<intervals>  SourceProductName=Simulink Design Verifier  SourceProductBaseCode=DV
  Relational Operator1 : RelationalOperator  RequirementInfo={} %GIDa_a961d2d7_3efd_48da_9f20_2c071cba4ef9  Operator===  OutDataTypeStr=boolean  RndMeth=Nearest
  Relational Operator10 : RelationalOperator  RequirementInfo={} %GIDa_47718f7c_343e_4447_b8d1_6fc0722b0600  Operator===  OutDataTypeStr=boolean  RndMeth=Nearest
  Relational Operator11 : RelationalOperator  RequirementInfo={} %GIDa_efafd513_65b0_4f45_b8c3_fc57da6567f0  Operator===  OutDataTypeStr=boolean  RndMeth=Nearest
  Relational Operator12 : RelationalOperator  RequirementInfo={} %GIDa_8351859b_929a_4cd6_92b1_a7bb9f964c4c  Operator===  OutDataTypeStr=boolean  RndMeth=Nearest
  Relational Operator13 : RelationalOperator  RequirementInfo={} %GIDa_b2e2f2ec_c0e5_4039_98ad_e792866cca98  Operator===  OutDataTypeStr=boolean  RndMeth=Nearest
  Relational Operator14 : RelationalOperator  RequirementInfo={} %GIDa_4dcbaae0_7e8f_4090_a75d_7fbbbbe3a3aa  Operator===  OutDataTypeStr=boolean  RndMeth=Nearest
  Relational Operator15 : RelationalOperator  RequirementInfo={} %GIDa_26deefd2_44bf_4401_8ea1_1f974cfdcafd  Operator===  OutDataTypeStr=boolean  RndMeth=Nearest
  Relational Operator16 : RelationalOperator  RequirementInfo={} %GIDa_caa90808_913a_4c34_ae1b_f934b0964348  Operator===  OutDataTypeStr=boolean  RndMeth=Nearest
  Relational Operator2 : RelationalOperator  RequirementInfo={} %GIDa_3f274450_fb8c_43b6_a1e1_021d4ca98f7a  Operator===  OutDataTypeStr=boolean  RndMeth=Nearest
  Relational Operator3 : RelationalOperator  RequirementInfo={} %GIDa_50c4d142_d821_4a0c_bdd0_9b403def1826  Operator===  OutDataTypeStr=boolean  RndMeth=Nearest
  Relational Operator4 : RelationalOperator  RequirementInfo={} %GIDa_e65f29f1_216a_4c97_b488_a5e50ac97795  Operator===  OutDataTypeStr=boolean  RndMeth=Nearest
  Relational Operator5 : RelationalOperator  RequirementInfo={} %GIDa_6010fb27_28a2_439c_8a99_657e11613bb6  Operator===  OutDataTypeStr=boolean  RndMeth=Nearest
  Relational Operator6 : RelationalOperator  RequirementInfo={} %GIDa_c2ccee74_c6cf_47fc_a1e0_8733f53042a1  Operator===  OutDataTypeStr=boolean  RndMeth=Nearest
  Relational Operator7 : RelationalOperator  RequirementInfo={} %GIDa_1118d708_063d_4a47_8656_57592d9dcdaf  Operator===  OutDataTypeStr=boolean  RndMeth=Nearest
  Relational Operator8 : RelationalOperator  RequirementInfo={} %GIDa_d4d21019_2395_431c_b20c_c75ed04f6317  Operator===  OutDataTypeStr=boolean  RndMeth=Nearest
  Relational Operator9 : RelationalOperator  RequirementInfo={} %GIDa_7b98f3df_90c5_4371_a5a5_9fc022c763c1  Operator===  OutDataTypeStr=boolean  RndMeth=Nearest
  Within Implies : sldvlib/Temporal Operators/Within Implies  RequirementInfo={} %GIDa_97d1e8ab_9aef_4e79_a7e0_e8c29c00ca3e  reset=off
      settings: SourceProductName=Simulink Design Verifier  SourceProductBaseCode=DV
  Within Implies1 : sldvlib/Temporal Operators/Within Implies  RequirementInfo={} %GIDa_419ac9b4_bc68_436b_bce1_509d752df669  reset=off
      settings: SourceProductName=Simulink Design Verifier  SourceProductBaseCode=DV
  Within Implies2 : sldvlib/Temporal Operators/Within Implies  RequirementInfo={} %GIDa_369d41fc_8ee1_4c9d_a1f9_96e81b17eb96  reset=off
      settings: SourceProductName=Simulink Design Verifier  SourceProductBaseCode=DV
  delayi1 : UnitDelay  RequirementInfo={} %GIDa_5f5c2eeb_4d25_4d43_8ef0_1e15d6d0f8b1  SampleTime=-1
  gte1 : RelationalOperator  RequirementInfo={} %GIDa_0e1d602c_88b0_4888_9dd6_22bd0e45e59a  OutDataTypeStr=boolean  RndMeth=Nearest
  wires:
  Delay10/1 -> Implies1/1
  Detector3/1 -> Delay10/1
  Relational Operator9/1 -> Implies1/2
  Delay8/1 -> Implies2/1
  Detector1/1 -> Delay8/1
  Relational Operator16/1 -> Implies2/2
  Constant12/1 -> Relational Operator10/2
  Relational Operator13/1 -> Logical Operator9/2
  Logical Operator8/1 -> Logical Operator10/1
  recoverable1/1 -> Relational Operator10/1
  Relational Operator14/1 -> Logical Operator8/2
  error1/1 -> Relational Operator14/1
  Implies2/1 -> Proof Objective5/1
  Relational Operator12/1 -> Logical Operator9/1
  Constant13/1 -> Relational Operator12/2
  Constant16/1 -> Relational Operator15/2
  Constant14/1 -> Relational Operator13/2
  Constant15/1 -> Relational Operator14/2
  Logical Operator9/1 -> Logical Operator8/1
  Logical Operator10/1 -> Detector1/1
  Relational Operator15/1 -> Logical Operator9/3
  Constant8/1 -> Relational Operator16/2
  stateFlowModeLS4/1 -> Relational Operator16/1, Relational Operator12/1, Relational Operator13/1, Relational Operator15/1
  Relational Operator10/1 -> Logical Operator10/2
  Constant10/1 -> Relational Operator9/2
  task_error/1 -> Relational Operator9/1
  Relational Operator11/1 -> Logical Operator7/2
  Logical Operator5/1 -> Logical Operator7/1
  Relational Operator7/1 -> Logical Operator5/2
  Constant7/1 -> Relational Operator7/2
  error/1 -> Relational Operator7/1
  Logical Operator6/1 -> Logical Operator5/1
  Relational Operator8/1 -> Logical Operator6/3
  Relational Operator5/1 -> Logical Operator6/2
  Relational Operator4/1 -> Logical Operator6/1
  Constant9/1 -> Relational Operator8/2
  Constant5/1 -> Relational Operator5/2
  Constant4/1 -> Relational Operator4/2
  stateFlowModeLS3/1 -> Relational Operator4/1, Relational Operator5/1, Relational Operator8/1
  Within Implies1/1 -> Proof Objective2/1
  Within Implies2/1 -> Proof Objective3/1
  Within Implies/1 -> Proof Objective1/1
  Logical Operator7/1 -> Detector3/1
  recoverable/1 -> Relational Operator11/1
  Constant11/1 -> Relational Operator11/2
  Implies1/1 -> Proof Objective4/1
  load_counter/1 -> Within Implies2/2
  Constant6/1 -> Relational Operator6/1
  stateFlowModeLS2/1 -> Relational Operator2/1, Relational Operator6/2
  Constant3/1 -> Relational Operator2/2
  Relational Operator2/1 -> Delay6/1
  Relational Operator6/1 -> Logical Operator4/1
  Delay6/1 -> Logical Operator4/2
  Logical Operator4/1 -> Within Implies2/1
  Delay3/1 -> Logical Operator2/1
  Logical Operator3/1 -> Within Implies1/1
  Logical Operator1/1 -> Within Implies1/2
  Delay/1 -> Delay1/1
  Delay4/1 -> Delay2/1
  Relational Operator1/1 -> Logical Operator3/1
  Logical Operator2/1 -> Logical Operator1/3
  Delay2/1 -> Logical Operator1/2
  Constant1/1 -> Relational Operator1/2
  Delay5/1 -> Delay/1
  ctrl1/1 -> Delay5/1, Delay3/1, Delay4/1
  Delay1/1 -> Logical Operator/1
  stateFlowModeLS1/1 -> Relational Operator1/1
  increment/1 -> Logical Operator3/2
  Logical Operator/1 -> Logical Operator1/1
  inst_ptr/1 -> gte1/1, delayi1/1
  stateFlowModeLS/1 -> Relational Operator3/1
  delayi1/1 -> gte1/2
  Constant2/1 -> Relational Operator3/2
  gte1/1 -> Within Implies/2
  Relational Operator3/1 -> Within Implies/1

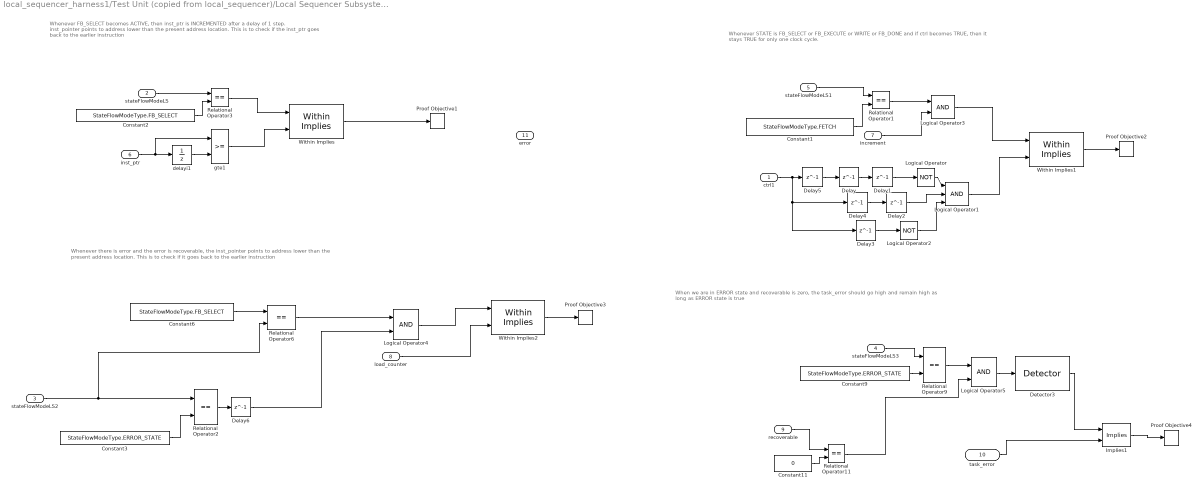
== system local_sequencer_harness1/Test Unit (copied from local_sequencer)/Local Sequencer Subsystem/Verification Subsystem1 ==
  note: When we are in ERROR state and recoverable is zero, the task_error should go high and remain high as
      | long as ERROR state is true
  note: Whenever there is error and the error is recoverable, the inst_pointer points to address lower than the present address location. This is to check if it goes back to the earlier instruction
  note: Whenever STATE is FB_SELECT or FB_EXECUTE or WRITE or FB_DONE and if ctrl becomes TRUE, then it stays TRUE for only one clock cycle.
  note: Whenever FB_SELECT becomes ACTIVE, then inst_ptr is INCREMENTED after a delay of 1 step. inst_pointer points to address lower than the present address location. This is to check if the inst_ptr goes back to the earlier instruction
  ctrl1 : Inport  RequirementInfo={} %GIDa_b2a8e237_8e08_4025_b16b_248d05a3ae4b
  stateFlowModeLS : Inport  RequirementInfo={} %GIDa_03d37cf9_993a_48b4_a09c_30bb73e5eb57  Port=2  OutDataTypeStr=Enum: StateFlowModeType
  stateFlowModeLS2 : Inport  RequirementInfo={} %GIDa_82246f40_cc55_428e_9123_699bef1aac57  Port=3  OutDataTypeStr=Enum: StateFlowModeType
  stateFlowModeLS3 : Inport  RequirementInfo={} %GIDa_b27ac389_dd1d_4ce1_9e3b_eb410def7c62  Port=4  OutDataTypeStr=Enum: StateFlowModeType
  stateFlowModeLS1 : Inport  RequirementInfo={} %GIDa_2aed1148_92aa_4fe6_972c_5d6e39105bb0  Port=5  OutDataTypeStr=Enum: StateFlowModeType
  inst_ptr : Inport  RequirementInfo={} %GIDa_2d5f27ad_ad32_4bbd_9ed8_0b6adf712739  Port=6
  increment : Inport  RequirementInfo={} %GIDa_9c2ad961_9799_4e16_af57_5bf5465648c3  Port=7
  load_counter : Inport  RequirementInfo={} %GIDa_d0c12f46_53aa_4d16_ad9d_3e9c55af9a8c  Port=8
  recoverable : Inport  RequirementInfo={} %GIDa_2b2f68b4_007b_4354_afb2_04c03372b7ee  Port=9
  task_error : Inport  RequirementInfo={} %GIDa_61a61786_5e77_465d_b091_51bd7d251149  Port=10
  error : Inport  RequirementInfo={} %GIDa_698ef9dc_bf00_41be_8f9e_4f87bd768571  Port=11
  Constant1 : Constant  RequirementInfo={} %GIDa_e25e3f7d_d174_4baa_824c_99dbb0a562c4  Value=StateFlowModeType.FETCH
  Constant11 : Constant  RequirementInfo={} %GIDa_dd5b5da3_c62a_4ca9_834b_daad37b36370  Value=0
  Constant2 : Constant  RequirementInfo={} %GIDa_7b350a3a_1e9d_44fa_851e_4f0b03332757  Value=StateFlowModeType.FB_SELECT
  Constant3 : Constant  RequirementInfo={} %GIDa_402dd0e2_0fd8_42e1_a1ed_1de159629a53  Value=StateFlowModeType.ERROR_STATE
  Constant6 : Constant  RequirementInfo={} %GIDa_f45152c4_2060_4ca9_8ea7_8cb2ccad9acb  Value=StateFlowModeType.FB_SELECT
  Constant9 : Constant  RequirementInfo={} %GIDa_29c53103_c422_4e21_bbe3_d5f691d38ac6  Value=StateFlowModeType.ERROR_STATE
  Delay : Delay  RequirementInfo={} %GIDa_659eef15_6fad_4f22_83b2_5a4fa9897b4c  DelayLength=1  InitialCondition=0
  Delay1 : Delay  RequirementInfo={} %GIDa_520b59dc_4130_43fd_a005_7459da35187e  DelayLength=1  InitialCondition=0
  Delay2 : Delay  RequirementInfo={} %GIDa_6fb618e8_15ef_4933_a5fd_f3f12513ba67  DelayLength=1  InitialCondition=0
  Delay3 : Delay  RequirementInfo={} %GIDa_f9ff44e2_8463_4b1a_8fb3_08e94bbb7bb7  DelayLength=1  InitialCondition=0
  Delay4 : Delay  RequirementInfo={} %GIDa_3128362c_4a52_4b5f_a166_4c99eed2aa87  DelayLength=1  InitialCondition=0
  Delay5 : Delay  RequirementInfo={} %GIDa_04c9a826_7518_43bb_b475_870918c73754  DelayLength=1  InitialCondition=0
  Delay6 : Delay  RequirementInfo={} %GIDa_6769fc34_2c8a_4fa2_8f4f_0ef2da45cbaa  DelayLength=1  InitialCondition=0
  Detector3 : sldvlib/Temporal Operators/Detector  RequirementInfo={} %GIDa_24979acb_1800_41d5_a6a8_74a2fa5f04e2  reset=off  typ=Synchronized  in_hold=1  delay=0  out_hold=5
      settings: SourceProductName=Simulink Design Verifier  SourceProductBaseCode=DV
  Implies1 : sldvlib/Verification Utilities/Implies  RequirementInfo={} %GIDa_0fb0e97f_40f0_4cab_9d94_882e74dab2a4
      settings: SourceProductName=Simulink Design Verifier  SourceProductBaseCode=DV
  Logical Operator : Logic  RequirementInfo={} %GIDa_58a59343_bc2b_47dc_8b72_4d0bdbe4f993  Operator=NOT  AllPortsSameDT=off  OutDataTypeStr=boolean
  Logical Operator1 : Logic  RequirementInfo={} %GIDa_fa70ff33_c249_47d3_bc1b_7b3b033c6391  Inputs=3  AllPortsSameDT=off  OutDataTypeStr=boolean
  Logical Operator2 : Logic  RequirementInfo={} %GIDa_2ff9253e_9991_4648_8ff1_1a0b6ee97db2  Operator=NOT  AllPortsSameDT=off  OutDataTypeStr=boolean
  Logical Operator3 : Logic  RequirementInfo={} %GIDa_12b0f31a_3d57_452f_98ab_bb273fe9e707  AllPortsSameDT=off  OutDataTypeStr=boolean
  Logical Operator4 : Logic  RequirementInfo={} %GIDa_e9250b2a_3a22_4342_b9fb_2902c9631241  AllPortsSameDT=off  OutDataTypeStr=boolean
  Logical Operator5 : Logic  RequirementInfo={} %GIDa_a9f46be8_c492_4761_a63a_a555ba9a23fb  AllPortsSameDT=off  OutDataTypeStr=boolean
  Proof Objective1 : sldvlib/Objectives and Constraints/Proof Objective  RequirementInfo={} %GIDa_50b1438d_6829_4c16_85f3_30667a64241b  enabled=on  customAVTBlockType=Proof Objective  intervals=true  dispValues=on  outEnabled=off  enableStopSim=off
      settings: AttributesFormatString=%<intervals>  SourceProductName=Simulink Design Verifier  SourceProductBaseCode=DV
  Proof Objective2 : sldvlib/Objectives and Constraints/Proof Objective  RequirementInfo={} %GIDa_d1bbe62a_0820_4344_a64d_edf0b2ccbf31  enabled=on  customAVTBlockType=Proof Objective  intervals=true  dispValues=on  outEnabled=off  enableStopSim=off
      settings: AttributesFormatString=%<intervals>  SourceProductName=Simulink Design Verifier  SourceProductBaseCode=DV
  Proof Objective3 : sldvlib/Objectives and Constraints/Proof Objective  RequirementInfo={} %GIDa_5f5fe716_a012_4cb1_bb0e_4a3e468a99d0  enabled=on  customAVTBlockType=Proof Objective  intervals=true  dispValues=on  outEnabled=off  enableStopSim=off
      settings: AttributesFormatString=%<intervals>  SourceProductName=Simulink Design Verifier  SourceProductBaseCode=DV
  Proof Objective4 : sldvlib/Objectives and Constraints/Proof Objective  RequirementInfo={} %GIDa_e53fd8ab_2635_432a_901f_7aa3a378c9e0  enabled=on  customAVTBlockType=Proof Objective  intervals=true  dispValues=on  outEnabled=off  enableStopSim=off
      settings: AttributesFormatString=%<intervals>  SourceProductName=Simulink Design Verifier  SourceProductBaseCode=DV
  Relational Operator1 : RelationalOperator  RequirementInfo={} %GIDa_13e594b6_4918_4e13_8086_ca82f7500aef  Operator===  OutDataTypeStr=boolean  RndMeth=Nearest
  Relational Operator11 : RelationalOperator  RequirementInfo={} %GIDa_7a461b09_85bc_48d8_9b7c_67a8d512599a  Operator===  OutDataTypeStr=boolean  RndMeth=Nearest
  Relational Operator2 : RelationalOperator  RequirementInfo={} %GIDa_566a4ac3_d50a_4cd1_8c71_84e9ed6612ac  Operator===  OutDataTypeStr=boolean  RndMeth=Nearest
  Relational Operator3 : RelationalOperator  RequirementInfo={} %GIDa_515f5bc9_39b1_4ce8_a94a_8beed421b585  Operator===  OutDataTypeStr=boolean  RndMeth=Nearest
  Relational Operator6 : RelationalOperator  RequirementInfo={} %GIDa_3e154368_6cff_44f9_bd9f_17b97fbd8727  Operator===  OutDataTypeStr=boolean  RndMeth=Nearest
  Relational Operator9 : RelationalOperator  RequirementInfo={} %GIDa_0b38a899_2c56_4293_906e_2cc9ba6059a3  Operator===  OutDataTypeStr=boolean  RndMeth=Nearest
  Within Implies : sldvlib/Temporal Operators/Within Implies  RequirementInfo={} %GIDa_ca53895a_8d60_4a5a_87b6_0e714fe95afe  reset=off
      settings: SourceProductName=Simulink Design Verifier  SourceProductBaseCode=DV
  Within Implies1 : sldvlib/Temporal Operators/Within Implies  RequirementInfo={} %GIDa_8d40f727_94d6_449d_b73b_b2b08665b8e5  reset=off
      settings: SourceProductName=Simulink Design Verifier  SourceProductBaseCode=DV
  Within Implies2 : sldvlib/Temporal Operators/Within Implies  RequirementInfo={} %GIDa_5bec92b2_7e6a_4dda_8e3e_90cd73e0f4f1  reset=off
      settings: SourceProductName=Simulink Design Verifier  SourceProductBaseCode=DV
  delayi1 : UnitDelay  RequirementInfo={} %GIDa_c259b9db_b4f2_49e4_9d6f_fa9eb7d108dc  SampleTime=-1
  gte1 : RelationalOperator  RequirementInfo={} %GIDa_66dfca42_481c_4672_aaa0_86cc52879db4  OutDataTypeStr=boolean  RndMeth=Nearest
  wires:
  Within Implies1/1 -> Proof Objective2/1
  Within Implies2/1 -> Proof Objective3/1
  Within Implies/1 -> Proof Objective1/1
  Detector3/1 -> Implies1/1
  Logical Operator5/1 -> Detector3/1
  Relational Operator11/1 -> Logical Operator5/2
  recoverable/1 -> Relational Operator11/1
  Constant11/1 -> Relational Operator11/2
  Relational Operator9/1 -> Logical Operator5/1
  task_error/1 -> Implies1/2
  Implies1/1 -> Proof Objective4/1
  Constant9/1 -> Relational Operator9/2
  stateFlowModeLS3/1 -> Relational Operator9/1
  load_counter/1 -> Within Implies2/2
  Constant6/1 -> Relational Operator6/1
  stateFlowModeLS2/1 -> Relational Operator2/1, Relational Operator6/2
  Constant3/1 -> Relational Operator2/2
  Relational Operator2/1 -> Delay6/1
  Relational Operator6/1 -> Logical Operator4/1
  Delay6/1 -> Logical Operator4/2
  Logical Operator4/1 -> Within Implies2/1
  Delay3/1 -> Logical Operator2/1
  Logical Operator3/1 -> Within Implies1/1
  Logical Operator1/1 -> Within Implies1/2
  Delay/1 -> Delay1/1
  Delay4/1 -> Delay2/1
  Relational Operator1/1 -> Logical Operator3/1
  Logical Operator2/1 -> Logical Operator1/3
  Delay2/1 -> Logical Operator1/2
  Constant1/1 -> Relational Operator1/2
  Delay5/1 -> Delay/1
  ctrl1/1 -> Delay5/1, Delay3/1, Delay4/1
  Delay1/1 -> Logical Operator/1
  stateFlowModeLS1/1 -> Relational Operator1/1
  increment/1 -> Logical Operator3/2
  Logical Operator/1 -> Logical Operator1/1
  inst_ptr/1 -> gte1/1, delayi1/1
  stateFlowModeLS/1 -> Relational Operator3/1
  delayi1/1 -> gte1/2
  Constant2/1 -> Relational Operator3/2
  gte1/1 -> Within Implies/2
  Relational Operator3/1 -> Within Implies/1
